simulink model "simulation"  (R2023a)
settings: Solver=VariableStepAuto  StartTime=0.0  StopTime=10.0  RelTol=1e-3
settings Model: Creator=dhruva  LastModifiedBy=dhruva

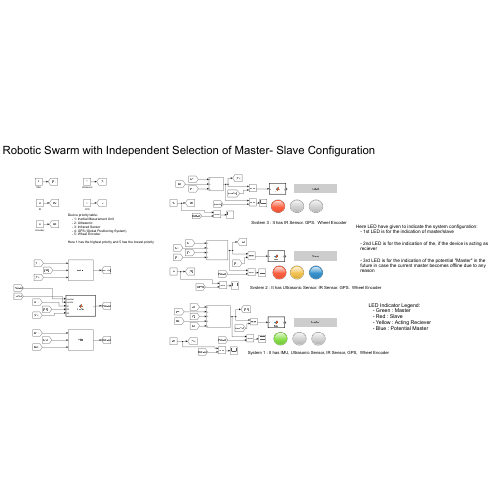
[thumbnail: Simulink's stored preview of the top-level diagram]
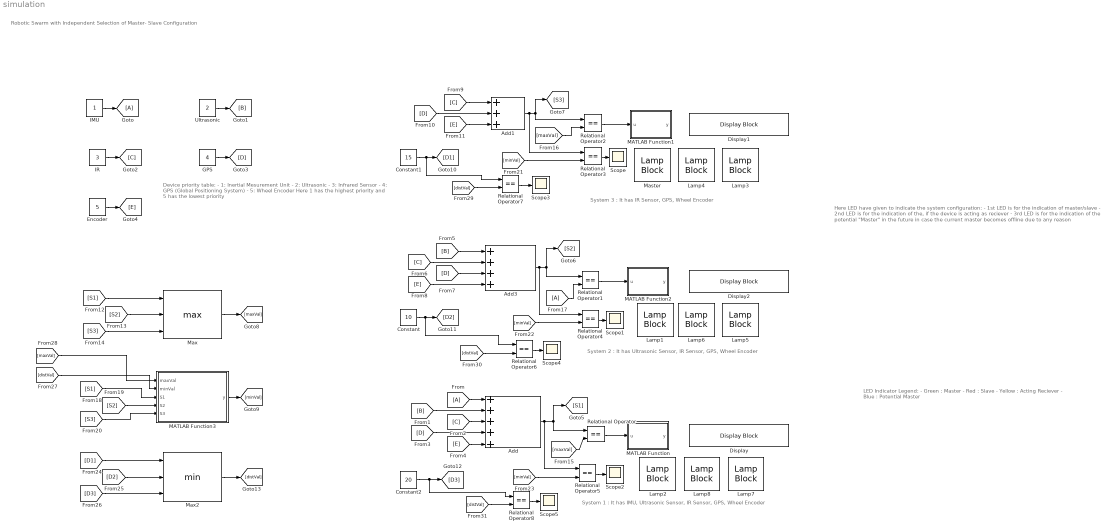
== system simulation ==
  note: LED Indicator Legend:
      | - Green : Master
      | - Red : Slave
      | - Yellow : Acting Reciever
      | - Blue : Potential Master
  note: Here LED have given to indicate the system configuration:
      | - 1st LED is for the indication of master/slave
      |
      | - 2nd LED is for the indication of the, if the device is acting as reciever
      |
      | - 3rd LED is for the indication of the potential "Master" in the future in case the current master becomes offline due to any reason
  note: System 1 : It has IMU, Ultrasonic Sensor, IR Sensor, GPS, Wheel Encoder
  note: Device priority table:
      | - 1: Inertial Mesurement Unit
      | - 2: Ultrasonic
      | - 3: Infrared Sensor
      | - 4: GPS (Global Positioning System)
      | - 5: Wheel Encoder
      |
      | Here 1 has the highest priority and 5 has the lowest priority
  note: Robotic Swarm with Independent Selection of Master- Slave Configuration
  note: System 2 : It has Ultrasonic Sensor, IR Sensor, GPS, Wheel Encoder
  note: System 3 : It has IR Sensor, GPS, Wheel Encoder
  Add : Sum  Inputs=+++++
  Add1 : Sum  Inputs=+++
  Add3 : Sum  Inputs=++++
  Constant : Constant  Value=10
  Constant1 : Constant  Value=15
  Constant2 : Constant  Value=20
  Display : DisplayBlock  LabelPosition=Hide  Transparency=1
  Display1 : DisplayBlock  LabelPosition=Hide  Transparency=1
  Display2 : DisplayBlock  LabelPosition=Hide  Transparency=1
  Encoder : Constant  Value=5
  From : From
  From17 : From
  GPS : Constant  Value=4
  Goto : Goto
  IMU : Constant
  IR : Constant  Value=3
  Lamp{1..8} (8 alike) : LampBlock  LabelPosition=Hide
  MATLAB Function : MATLAB Function  TreatAsAtomicUnit=on
  MATLAB Function1 : MATLAB Function  TreatAsAtomicUnit=on
  MATLAB Function2 : MATLAB Function  TreatAsAtomicUnit=on
  MATLAB Function3 : MATLAB Function  TreatAsAtomicUnit=on
  Master : LampBlock  LabelPosition=Hide
  Max : MinMax  Function=max  Inputs=3
  Max2 : MinMax  Inputs=3
  Relational Operator{,1..8} (9 alike) : RelationalOperator  Operator===  OutDataTypeStr=boolean  RndMeth=Simplest  InputSameDT=off
  Scope{,1..5} (6 alike) : Scope
  Ultrasonic : Constant  Value=2
  wires:
  IMU/1 -> Goto/1
  Ultrasonic/1 -> [B]
  IR/1 -> [C]
  GPS/1 -> [D]
  Encoder/1 -> [E]
  From/1 -> Add/1
  [B] -> Add/2
  [C] -> Add/3
  [D] -> Add/4
  [E] -> Add/5
  [B] -> Add3/1
  [C] -> Add3/2
  [D] -> Add3/3
  [E] -> Add3/4
  [C] -> Add1/1
  [D] -> Add1/2
  [E] -> Add1/3
  Add/1 -> Relational Operator5/1, Relational Operator/1, [S1]
  Add3/1 -> Relational Operator4/1, Relational Operator1/1, [S2]
  Add1/1 -> Relational Operator3/1, Relational Operator2/1, [S3]
  [S1] -> Max/1
  [S2] -> Max/2
  [S3] -> Max/3
  [maxVal] -> Relational Operator/2
  Max/1 -> [maxVal]
  Relational Operator/1 -> MATLAB Function/1(u)
  [maxVal] -> Relational Operator2/2
  Relational Operator2/1 -> MATLAB Function1/1(u)
  From17/1 -> Relational Operator1/2
  Relational Operator1/1 -> MATLAB Function2/1(u)
  Relational Operator4/1 -> Scope1/1
  [minVal] -> Relational Operator3/2
  [minVal] -> Relational Operator4/2
  Relational Operator3/1 -> Scope/1
  [minVal] -> Relational Operator5/2
  Relational Operator5/1 -> Scope2/1
  Constant1/1 -> Relational Operator7/1, [D1]
  Constant/1 -> Relational Operator6/1, [D2]
  Constant2/1 -> Relational Operator8/1, [D3]
  Max2/1 -> [distVal]
  [D3] -> Max2/3
  [D2] -> Max2/2
  [D1] -> Max2/1
  [S3] -> MATLAB Function3/5(S3)
  [S2] -> MATLAB Function3/4(S2)
  [S1] -> MATLAB Function3/3(S1)
  [maxVal] -> MATLAB Function3/1(maxVal)
  [distVal] -> MATLAB Function3/2(minVal)
  MATLAB Function3/1(y) -> [minVal]
  [distVal] -> Relational Operator7/2
  [distVal] -> Relational Operator6/2
  [distVal] -> Relational Operator8/2
  Relational Operator7/1 -> Scope3/1
  Relational Operator6/1 -> Scope4/1
  Relational Operator8/1 -> Scope5/1

== matlab function simulation/MATLAB Function1 ==
  data: u input; y output
function y = fcn1(u)
if u
    y = "Master";
else
    y = "Slave";
end

== matlab function simulation/MATLAB Function ==
  data: u input; y output
function y = fcn(u)
if u
    y = "Master";
else
    y = "Slave";
end

== matlab function simulation/MATLAB Function2 ==
  data: u input; y output
function y = fcn(u)
if u
    y = "Master";
else
    y = "Slave";
end

== matlab function simulation/MATLAB Function3 ==
  data: maxVal input; y output; minVal input; S1 input; S2 input; S3 input
function y = fcn56(maxVal, minVal, S1, S2, S3)
if S1 ~= maxVal && S1 ~=minVal 
    y = S1;
elseif S2 ~= maxVal && S2 ~=minVal
    y = S2;
else
    y = S3;
end
